simulink model "Unmodel_Dynamics_Ex17"  (R2023a)
settings: Solver=VariableStepAuto  StartTime=0.0  StopTime=30.0  RelTol=1e-3
undefined symbols (not defined in the file): a, b, gamma1, gamma2, mi, sigma, ti
settings Model: Creator=geokr  LastModifiedBy=geokr

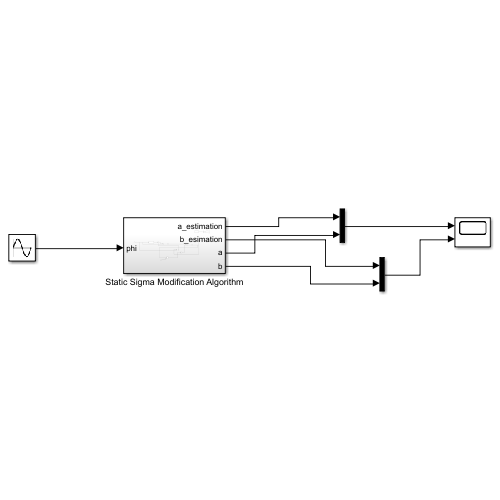
[thumbnail: Simulink's stored preview of the top-level diagram]
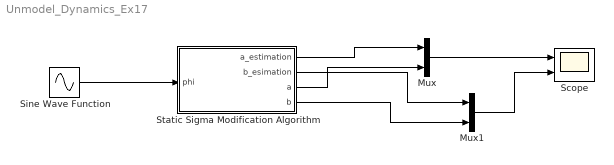
== system Unmodel_Dynamics_Ex17 ==
  Mux : Mux  Inputs=2
  Mux1 : Mux  Inputs=2
  Scope : Scope  NumInputPorts=2
  Sine Wave Function : Sin  Amplitude=4  Frequency=2  SampleTime=0
  Static Sigma Modification Algorithm : Subsystem
  wires:
  Sine Wave Function/1 -> Static Sigma Modification Algorithm/1(phi)
  Static Sigma Modification Algorithm/2(b_esimation) -> Mux1/1
  Static Sigma Modification Algorithm/4(b) -> Mux1/2
  Static Sigma Modification Algorithm/1(a_estimation) -> Mux/1
  Static Sigma Modification Algorithm/3(a) -> Mux/2
  Mux/1 -> Scope/1
  Mux1/1 -> Scope/2

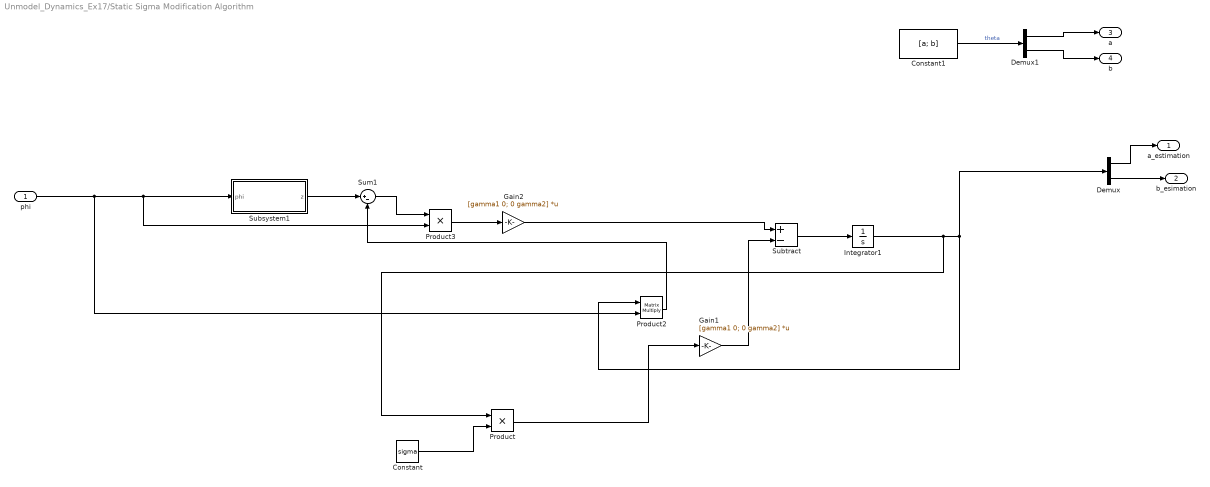
== system Unmodel_Dynamics_Ex17/Static Sigma Modification Algorithm ==
  phi : Inport
  Constant : Constant  Value=sigma
  Constant1 : Constant  Value=[a; b]  VectorParams1D=off
  Demux : Demux  Outputs=2
  Demux1 : Demux  Outputs=2
  Gain1 : Gain  Gain=[gamma1 0; 0 gamma2]  Multiplication=Matrix(K*u)
  Gain2 : Gain  Gain=[gamma1 0; 0 gamma2]  Multiplication=Matrix(K*u)
  Integrator1 : Integrator
  Product : Product
  Product2 : Product  Multiplication=Matrix(*)
  Product3 : Product
  Subsystem1 : Subsystem
  Subtract : Sum  Inputs=+-
  Sum1 : Sum  Inputs=|+-
  a_estimation : Outport
  b_esimation : Outport  Port=2
  a : Outport  Port=3
  b : Outport  Port=4
  wires:
  Subsystem1/1(z) -> Sum1/1
  Product2/1 -> Sum1/2
  Product3/1 -> Gain2/1
  phi/1 -> Subsystem1/1(phi), Product3/2, Product2/2
  Sum1/1 -> Product3/1
  Gain2/1 -> Subtract/1
  Subtract/1 -> Integrator1/1
  Gain1/1 -> Subtract/2
  Integrator1/1 -> Product/1, Demux/1, Product2/1
  Constant/1 -> Product/2
  Product/1 -> Gain1/1
  Constant1/1 -> Demux1/1  "theta"
  Demux/1 -> a_estimation/1
  Demux/2 -> b_esimation/1
  Demux1/1 -> a/1
  Demux1/2 -> b/1

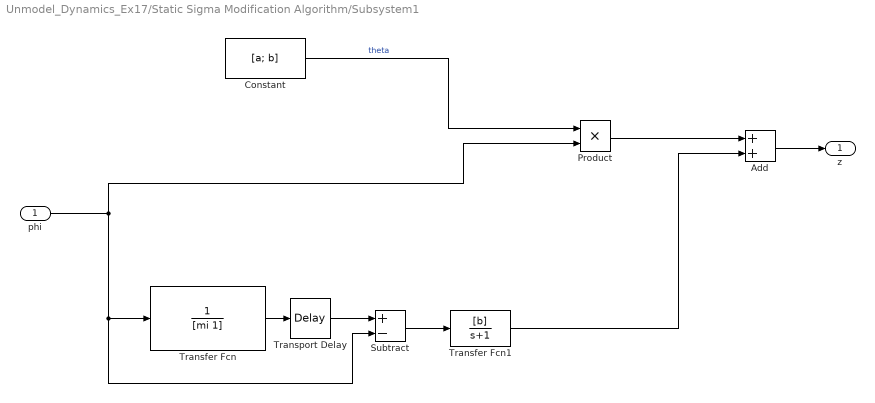
== system Unmodel_Dynamics_Ex17/Static Sigma Modification Algorithm/Subsystem1 ==
  phi : Inport
  Add : Sum
  Constant : Constant  Value=[a; b]  VectorParams1D=off
  Product : Product
  Subtract : Sum  Inputs=+-
  Transfer Fcn : TransferFcn  Denominator=[mi 1]
  Transfer Fcn1 : TransferFcn  Numerator=[b]  Denominator=[1 1]
  Transport Delay : TransportDelay  DelayTime=ti
  z : Outport
  wires:
  Constant/1 -> Product/1  "theta"
  Product/1 -> Add/1
  Add/1 -> z/1
  Transfer Fcn/1 -> Transport Delay/1
  Transport Delay/1 -> Subtract/1
  Subtract/1 -> Transfer Fcn1/1
  Transfer Fcn1/1 -> Add/2
  phi/1 -> Product/2, Transfer Fcn/1, Subtract/2
